simulink model "ex_3_sim"  (R2024b)
settings: Solver=VariableStepAuto  StartTime=0.0  StopTime=20  FixedStep=Ts  RelTol=1e-3
values from neighbouring files (symbols this model uses):
  A = [0, 1; -2, -40]    [Script.m]
  B = [0; 40]    [Script.m]
  C = [1, 0]    [Script.m]
  D = 0    [Script.m]
  Gamma_obs = [Gamma, L]    [Script.m]
  H_obs = eye(n)    [Script.m]
  J_obs = zeros(n, m+p)    [Script.m]
  K = Kz(2:end)    [Script.m]
  Ki = Kz(1)    [Script.m]
  Nu = sol(n+1:end)    [Script.m]
  Nx = sol(1:n)    [Script.m]
  Phi_obs = Phi-L*H    [Script.m]
  Ts = 0.01e-3    (= 1e-05)    [Script.m]
undefined symbols (not defined in the file or in its folder): DiscIntNeverNeededParam
settings Model: Creator=andre  LastModifiedBy=Enrico 2

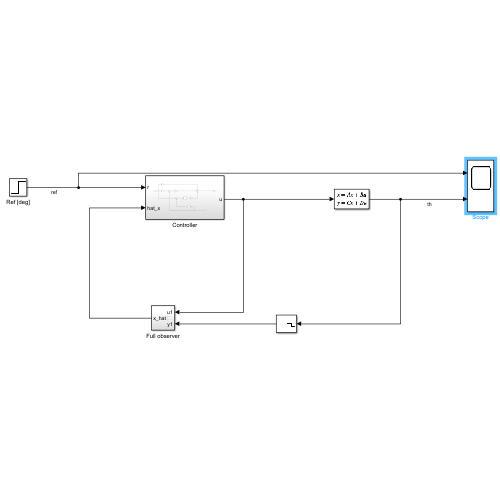
[thumbnail: Simulink's stored preview of the top-level diagram]
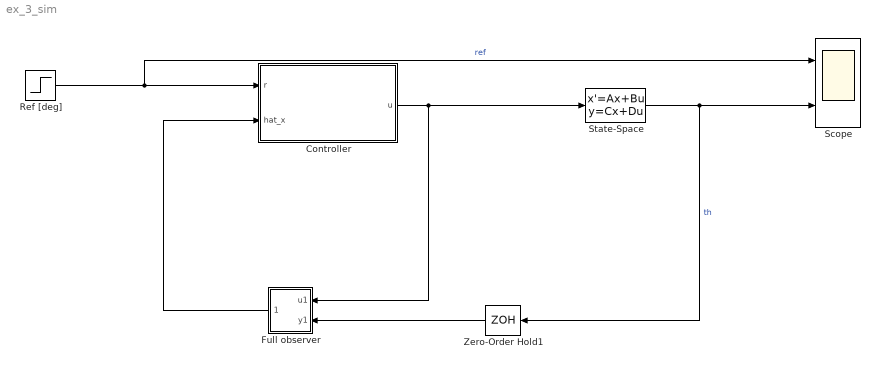
== system ex_3_sim ==
  Controller : Subsystem
  Full observer : Subsystem
  Ref [deg] : Step  After=100  SampleTime=0
  Scope : Scope  NumInputPorts=2
  State-Space : StateSpace  A=A  B=B  C=C  D=D  InitialCondition=0
  Zero-Order Hold1 : ZeroOrderHold  SampleTime=Ts
  wires:
  State-Space/1 -> Scope/2, Zero-Order Hold1/1  "th"
  Zero-Order Hold1/1 -> Full observer/2(y1)
  Ref [deg]/1 -> Scope/1, Controller/1(r)  "ref"
  Full observer/1(x_hat) -> Controller/2(hat_x)
  Controller/1(u) -> State-Space/1, Full observer/1(u1)

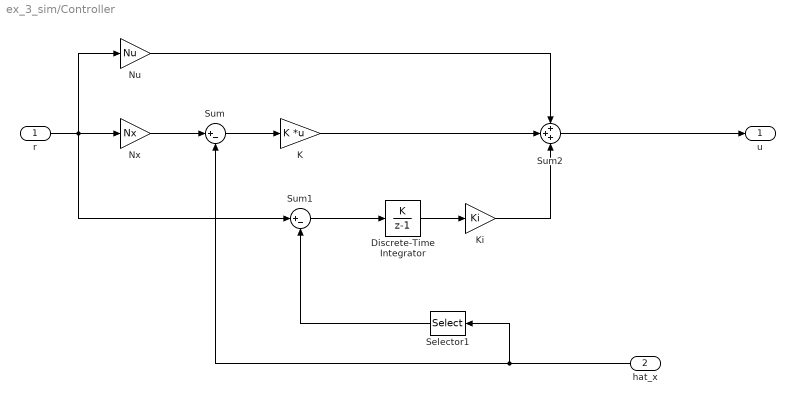
== system ex_3_sim/Controller ==
  r : Inport
  hat_x : Inport  Port=2
  Discrete-Time Integrator : DiscreteIntegrator  IntegratorMethod=Accumulation: Forward Euler  SampleTime=Ts  ICPrevOutput=DiscIntNeverNeededParam  ICPrevScaledInput=DiscIntNeverNeededParam
  K : Gain  Gain=K  Multiplication=Matrix(K*u)
  Ki : Gain  Gain=Ki
  Nu : Gain  Gain=Nu
  Nx : Gain  Gain=Nx
  Selector1 : Selector  InputPortWidth=2  IndexOptions=Index vector (dialog)  Indices=1  OutputSizes=1
  Sum : Sum  Inputs=|+-
  Sum1 : Sum  Inputs=|+-
  Sum2 : Sum  Inputs=+++
  u : Outport
  wires:
  K/1 -> Sum2/2
  Sum1/1 -> Discrete-Time Integrator/1
  Sum2/1 -> u/1
  Sum/1 -> K/1
  Nu/1 -> Sum2/1
  Selector1/1 -> Sum1/2
  hat_x/1 -> Selector1/1, Sum/2
  Ki/1 -> Sum2/3
  Nx/1 -> Sum/1
  r/1 -> Sum1/1, Nu/1, Nx/1
  Discrete-Time Integrator/1 -> Ki/1

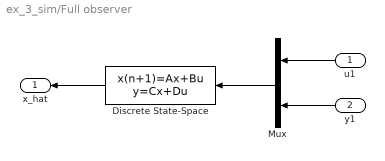
== system ex_3_sim/Full observer ==
  u1 : Inport
  y1 : Inport  Port=2
  Discrete State-Space : DiscreteStateSpace  A=Phi_obs  B=Gamma_obs  C=H_obs  D=J_obs  SampleTime=Ts
  Mux : Mux  Inputs=2
  x_hat : Outport
  wires:
  Discrete State-Space/1 -> x_hat/1
  Mux/1 -> Discrete State-Space/1
  y1/1 -> Mux/2
  u1/1 -> Mux/1
